simulink model "test"  (R2018a)
settings: Solver=FixedStepAuto  StartTime=0.0  StopTime=10.0  FixedStep=0.002  RelTol=1e-3
values from neighbouring files (symbols this model uses):
  ae1 = 1.3623    [bvp4c_helo.m]    (also in bvp4c_heloNEW.m = 1.3969; bvp4c_heloNEW2.m = 1.3969; opt_trajectory_SP_v2.m)
  ae2 = -0.3787    [bvp4c_helo.m]    (also in bvp4c_heloNEW.m = -0.1037; bvp4c_heloNEW2.m = -0.1037; opt_trajectory_SP_v2.m)
  at = -0.4638    [bvp4c_helo.m]    (also in bvp4c_heloNEW.m = -0.2032; bvp4c_heloNEW2.m = -0.2032; opt_trajectory_SP_v2.m)
  be = 0.1163    [bvp4c_helo.m]    (also in bvp4c_heloNEW.m = 0.3502; bvp4c_heloNEW2.m = 0.3502; opt_trajectory_SP_v2.m)
  bl = -0.1032    [bvp4c_helo.m]    (also in bvp4c_heloNEW.m = 0.2915; bvp4c_heloNEW2.m = 0.2915; opt_trajectory_SP_v2.m)
  bt = 0.9621    [bvp4c_helo.m]    (also in bvp4c_heloNEW.m = 1.9707; bvp4c_heloNEW2.m = 1.9707; opt_trajectory_SP_v2.m)
  ce = 0.0447    [bvp4c_helo.m]    (also in bvp4c_heloNEW.m = 0.2642; bvp4c_heloNEW2.m = 0.2642; opt_trajectory_SP_v2.m)
  cl = 0.2025    [bvp4c_helo.m]    (also in bvp4c_heloNEW.m = 0.0174; bvp4c_heloNEW2.m = 0.0174; opt_trajectory_SP_v2.m)
  ct = 0.0076    [bvp4c_helo.m]    (also in bvp4c_heloNEW.m = 0.4579; bvp4c_heloNEW2.m = 0.4579; opt_trajectory_SP_v2.m)
  x0 = [0;0;0;0;0;0]    [opt_trajectory_SP_v2.m]
settings Model: Creator=chirtsov  LastModifiedBy=chirtsov

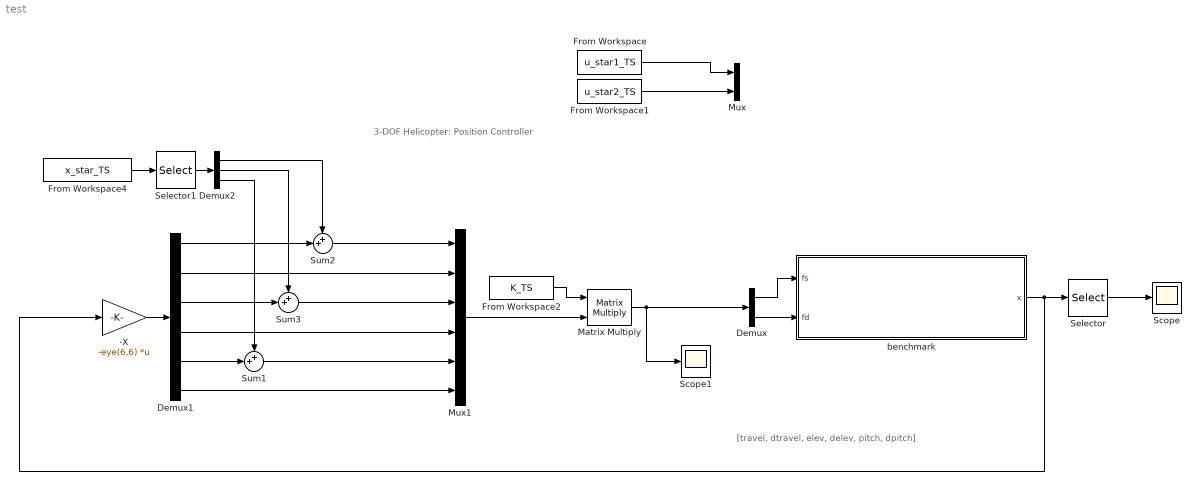
== system test ==
  note: 3-DOF Helicopter: Position Controller
  note: [travel, dtravel, elev, delev, pitch, dpitch]
  -X : Gain  Gain=-eye(6,6)  Multiplication=Matrix(K*u)
  Demux : Demux  Outputs=2
  Demux1 : Demux  Outputs=6
  Demux2 : Demux  Outputs=3
  From Workspace : FromWorkspace  VariableName=u_star1_TS  SampleTime=0
  From Workspace1 : FromWorkspace  VariableName=u_star2_TS  SampleTime=0
  From Workspace2 : FromWorkspace  VariableName=K_TS  SampleTime=0
  From Workspace4 : FromWorkspace  VariableName=x_star_TS  SampleTime=0
  Matrix Multiply : Product  Multiplication=Matrix(*)
  Mux : Mux  Inputs=2
  Mux1 : Mux  Inputs=6
  Scope : Scope
  Scope1 : Scope
  Selector : Selector  InputPortWidth=6  IndexOptions=Index vector (dialog)  Indices=[1 3 5]  OutputSizes=1
  Selector1 : Selector  InputPortWidth=6  IndexOptions=Index vector (dialog)  Indices=[1 3 5]  OutputSizes=1
  Sum1 : Sum  Inputs=++|
  Sum2 : Sum  Inputs=++|
  Sum3 : Sum  Inputs=++|
  benchmark : Subsystem
  wires:
  Selector/1 -> Scope/1
  From Workspace/1 -> Mux/1
  From Workspace1/1 -> Mux/2
  Matrix Multiply/1 -> Scope1/1, Demux/1
  Demux/1 -> benchmark/1("fs ")
  Demux/2 -> benchmark/2("fd ")
  Demux1/6 -> Mux1/6
  Sum2/1 -> Mux1/1
  benchmark/1(x) -> -X/1, Selector/1
  Demux1/2 -> Mux1/2
  Demux2/1 -> Sum2/1
  Sum3/1 -> Mux1/3
  From Workspace4/1 -> Selector1/1
  Demux1/1 -> Sum2/2
  Demux1/4 -> Mux1/4
  -X/1 -> Demux1/1
  Demux2/2 -> Sum3/1
  Demux1/3 -> Sum3/2
  Selector1/1 -> Demux2/1
  Demux1/5 -> Sum1/2
  Sum1/1 -> Mux1/5
  Demux2/3 -> Sum1/1
  From Workspace2/1 -> Matrix Multiply/1
  Mux1/1 -> Matrix Multiply/2

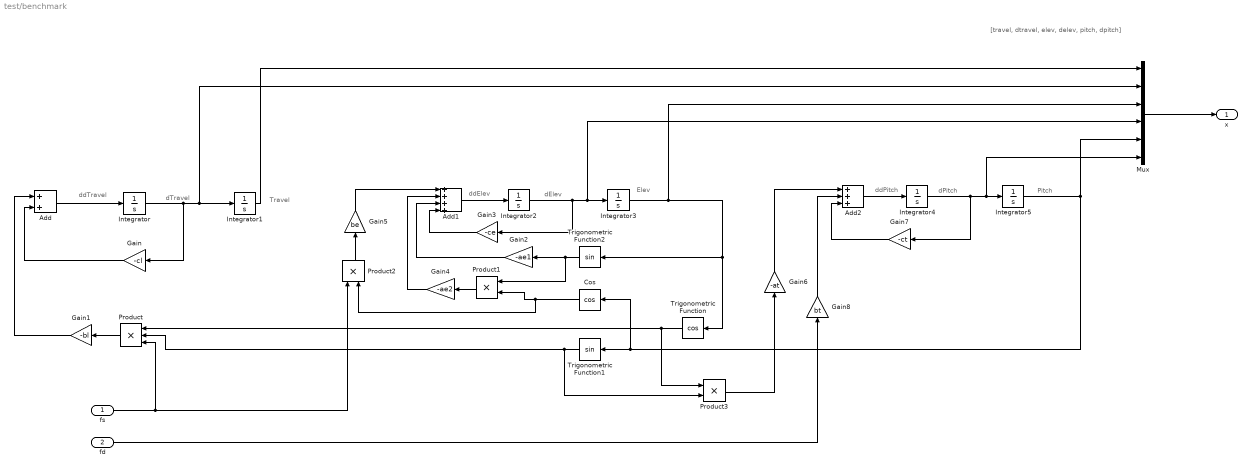
== system test/benchmark ==
  note: Pitch
  note: dPitch
  note: ddPitch
  note: Elev
  note: dElev
  note: ddElev
  note: Travel
  note: dTravel
  note: ddTravel
  note: [travel, dtravel, elev, delev, pitch, dpitch]
  "fs " : Inport
  "fd " : Inport  Port=2
  Add : Sum
  Add1 : Sum  Inputs=++++
  Add2 : Sum  Inputs=+++
  Cos : Trigonometry  Operator=cos
  Gain : Gain  Gain=-cl
  Gain1 : Gain  Gain=-bl
  Gain2 : Gain  Gain=-ae1
  Gain3 : Gain  Gain=-ce
  Gain4 : Gain  Gain=-ae2
  Gain5 : Gain  Gain=be
  Gain6 : Gain  Gain=-at
  Gain7 : Gain  Gain=-ct
  Gain8 : Gain  Gain=bt
  Integrator : Integrator  InitialCondition=x0(2)
  Integrator1 : Integrator  InitialCondition=x0(1)
  Integrator2 : Integrator  InitialCondition=x0(4)
  Integrator3 : Integrator  InitialCondition=x0(3)
  Integrator4 : Integrator  InitialCondition=x0(6)
  Integrator5 : Integrator  InitialCondition=x0(5)
  Mux : Mux  Inputs=6
  Product : Product  Inputs=3
  Product1 : Product
  Product2 : Product
  Product3 : Product
  Trigonometric Function : Trigonometry  Operator=cos
  Trigonometric Function1 : Trigonometry
  Trigonometric Function2 : Trigonometry
  x : Outport
  wires:
  Gain5/1 -> Add1/1
  Product/1 -> Gain1/1
  Product2/1 -> Gain5/1
  "fd "/1 -> Gain8/1
  Trigonometric Function/1 -> Product3/1, Product/1
  Product3/1 -> Gain6/1
  Gain7/1 -> Add2/3
  Cos/1 -> Product2/2, Product1/2
  Gain4/1 -> Add1/2
  Gain2/1 -> Add1/3
  Mux/1 -> x/1
  Gain8/1 -> Add2/2
  Add2/1 -> Integrator4/1
  Gain6/1 -> Add2/1
  Integrator1/1 -> Mux/1
  Gain1/1 -> Add/1
  Integrator3/1 -> Mux/3, Trigonometric Function2/1, Trigonometric Function/1
  Integrator2/1 -> Gain3/1, Mux/4, Integrator3/1
  Product1/1 -> Gain4/1
  Gain3/1 -> Add1/4
  Integrator4/1 -> Gain7/1, Mux/6, Integrator5/1
  Integrator/1 -> Gain/1, Mux/2, Integrator1/1
  Gain/1 -> Add/2
  Add1/1 -> Integrator2/1
  Integrator5/1 -> Mux/5, Cos/1, Trigonometric Function1/1
  Trigonometric Function2/1 -> Product1/1, Gain2/1
  Trigonometric Function1/1 -> Product3/2, Product/2
  "fs "/1 -> Product2/1, Product/3
  Add/1 -> Integrator/1
